simulink model "M_Kupfmullera"  (R2018a)
settings: Solver=VariableStepAuto  StartTime=0.0  StopTime=t  RelTol=1e-3
values from neighbouring files (symbols this model uses):
  k = 18.05    [model.m]
  tau2 = 280    [model.m]
  Tz = 580    [model.m]
  U = 0.95    [model.m]
settings Model: Creator=Kapi  LastModifiedBy=Kapi

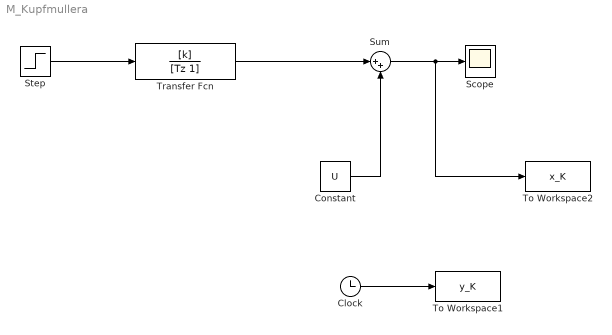
== system M_Kupfmullera ==
  Clock : Clock
  Constant : Constant  Value=U
  Scope : Scope
  Step : Step  Time=tau2  SampleTime=0
  Sum : Sum  Inputs=|++
  To Workspace1 : ToWorkspace  VariableName=y_K  SampleTime=-1
  To Workspace2 : ToWorkspace  VariableName=x_K  SampleTime=-1
  Transfer Fcn : TransferFcn  Numerator=[k]  Denominator=[Tz 1]
  wires:
  Step/1 -> Transfer Fcn/1
  Clock/1 -> To Workspace1/1
  Transfer Fcn/1 -> Sum/1
  Sum/1 -> To Workspace2/1, Scope/1
  Constant/1 -> Sum/2
